simulink subsystem "get_data_p_d_q_d_subsys"  (R2022b)
settings: Solver=VariableStepAuto  StartTime=0.0  StopTime=10.0  RelTol=1e-3
settings Model: Creator=emu  LastModifiedBy=rslstudent

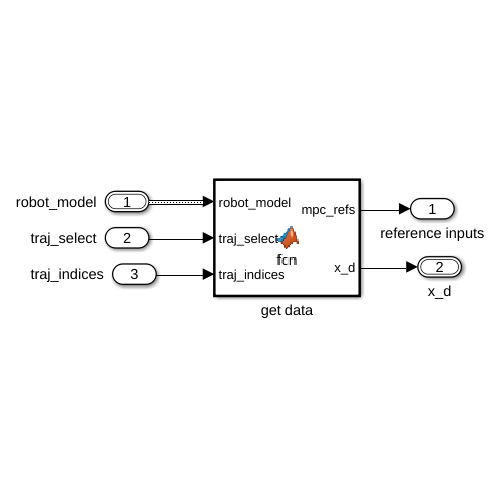
[thumbnail: Simulink's stored preview of the top-level diagram]
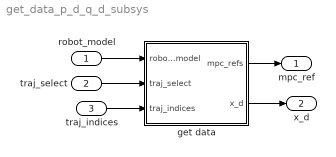
== system get_data_p_d_q_d_subsys ==
  robot_model : Inport  OutDataTypeStr=Bus: robot_model
  traj_select : Inport  Port=2
  traj_indices : Inport  Port=3
  get data : MATLAB Function  TreatAsAtomicUnit=on
  mpc_ref : Outport
  x_d : Outport  Port=2  OutDataTypeStr=Bus: x_d
  wires:
  get data/1(mpc_refs) -> mpc_ref/1
  traj_select/1 -> get data/2(traj_select)
  traj_indices/1 -> get data/3(traj_indices)
  get data/2(x_d) -> x_d/1
  robot_model/1 -> get data/1(robot_model)

== matlab function get_data_p_d_q_d_subsys/get data ==
  settings: updateMethod=DISCRETE  sampleTime=param_global.Ta
  data: mpc_refs output; robot_model input Bus: robot_model; traj_select input; param_traj_data parameter; traj_indices input; x_d output Bus: x_d
function [mpc_refs, x_d]  = fcn(robot_model, traj_select, param_traj_data, traj_indices)
persistent cnt;

if(isempty(cnt))
    cnt = 1;
end

traj_indices = traj_indices + (cnt-1);

% Parameters
q    = robot_model.q;      % generalized coordinates
q_p  = robot_model.q_p;  % time derivative of generalized coordinates

%{
x_k = [q;q_p];

% Assemble vector of recieved output measurements
p_d     = param_traj_data.p_d(   1:3, traj_indices, traj_select);
q_d     = param_traj_data.q_d(   1:4, traj_indices, traj_select);

y_d = [p_d; q_d];
%}

%%{
q_24_indices = [2 3]; % q2, q4 only (q3 ist deaktiviert daher ist q4 an index 3)
pos_indices = [1 3]; % xz plane

x_k = [q(q_24_indices);q_p(q_24_indices)];
p_d     = param_traj_data.p_d(   pos_indices, traj_indices, traj_select);
y_d = p_d;
%}

%% Reference out
mpc_refs = [x_k(:); y_d(:)];

%% Offline Trajectory out
x_d.p_d            = param_traj_data.p_d(           :,    cnt, traj_select);
x_d.p_d_p          = param_traj_data.p_d_p(         :,    cnt, traj_select);
x_d.p_d_pp         = param_traj_data.p_d_pp(        :,    cnt, traj_select);
x_d.Phi_d          = param_traj_data.Phi_d(         :,    cnt, traj_select);
x_d.Phi_d_p        = param_traj_data.Phi_d_p(       :,    cnt, traj_select);
x_d.Phi_d_pp       = param_traj_data.Phi_d_pp(      :,    cnt, traj_select);
x_d.R_d            = param_traj_data.R_d(           :, :, cnt, traj_select);
x_d.q_d            = param_traj_data.q_d(           :,    cnt, traj_select);
x_d.q_d_p          = param_traj_data.q_d_p(         :,    cnt, traj_select);
x_d.q_d_pp         = param_traj_data.q_d_pp(        :,    cnt, traj_select);
x_d.omega_d        = param_traj_data.omega_d(       :,    cnt, traj_select);
x_d.omega_d_p      = param_traj_data.omega_d_p(     :,    cnt, traj_select);
x_d.alpha_d        = param_traj_data.alpha_d(       :,    cnt, traj_select);
x_d.alpha_d_p      = param_traj_data.alpha_d_p(     :,    cnt, traj_select);
x_d.alpha_d_pp     = param_traj_data.alpha_d_pp(    :,    cnt, traj_select);
x_d.rot_ax_d       = param_traj_data.rot_ax_d(      :,    cnt, traj_select);
x_d.alpha_d_offset = param_traj_data.alpha_d_offset(:,    cnt, traj_select);
x_d.q_d_rel        = param_traj_data.q_d_rel(       :,    cnt, traj_select);

cnt = cnt+1;
